simulink subsystem "Controlador_BA"  (R2024b)
settings: Solver=VariableStepAuto  StartTime=0.0  StopTime=10.0  RelTol=1e-3
settings Model: Creator=Chenfu  LastModifiedBy=Chenfu

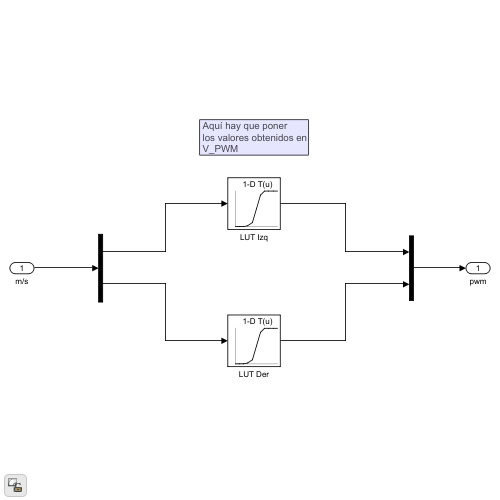
[thumbnail: Simulink's stored preview of the top-level diagram]
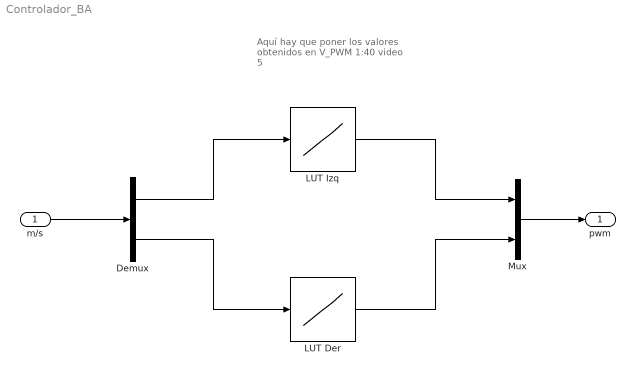
== system Controlador_BA ==
  note: Aquí hay que poner
      | los valores obtenidos en
      | V_PWM
      | 1:40 video 5
  m/s : Inport
  Demux : Demux  Outputs=2
  LUT Der : Lookup_n-D  NumberOfTableDimensions=1  BreakpointsForDimension1=[-5:5]  Table=tanh([-5:5])  InternalRulePriority=Speed  RndMeth=Simplest
  LUT Izq : Lookup_n-D  NumberOfTableDimensions=1  BreakpointsForDimension1=[-5:5]  Table=tanh([-5:5])  InternalRulePriority=Speed  RndMeth=Simplest
  Mux : Mux  Inputs=2
  pwm : Outport
  wires:
  m/s/1 -> Demux/1
  Demux/2 -> LUT Der/1
  Demux/1 -> LUT Izq/1
  LUT Izq/1 -> Mux/1
  LUT Der/1 -> Mux/2
  Mux/1 -> pwm/1
